simulink library "per"  (Simulink 8.2)
settings: Solver=ode45  StartTime=0.0  StopTime=10.0  RelTol=1e-3
undefined symbols (not defined in the file or in its folder): C_TICK_TIME_S, ENUM_LANEQUALITY_HIGH, ENUM_LANEQUALITY_MEDIUM, ENUM_SENSORSTATE_NORMAL, FALSE, KAPP_VehicleWidth_m, KPER_C0CrossingThr_m, KPER_CalDefaultTLC_s, KPER_CalTLCMax_s, KPER_CalTLCMin_s, KPER_DefaultLaneWidth_m, KPER_LaneWidHoldOnTime_s, KPER_LaneWidRampFinErrThres_m, KPER_LaneWidRampFinTimeThres_s, KPER_LaneWidRampInFalRt_mps, KPER_LaneWidRampInRisRt_mps, KPER_LaneWidRampOutFalRt_mps, KPER_LaneWidRampOutRisRt_mps, KPER_TLCDefaultValue_s, KPER_UseCalTLC_flg, TRUE
libraries: hcu_lib x16, cam x1, rad x1, sdf x1
(part 2 of 2)

== system per/PER/per/Lane_Process/LaneCalculation/GenerateRightLane ==
  VDINR_LaneC0R_m : Inport
  VPER_EstLaneC0R_m : Inport  Port=2
  VDINR_LaneC1R_rad : Inport  Port=3
  VPER_EstLaneC1R_rad : Inport  Port=4
  VDINR_LaneC2R_rat : Inport  Port=5
  VPER_EstLaneC2R_rat : Inport  Port=6
  VDINR_LaneC3R_rat : Inport  Port=7
  VPER_EstLaneC3R_rat : Inport  Port=8
  VPER_RightLaneAvail_flg : Inport  Port=9
  Switch{3,12..14} (4 alike) : Switch  Criteria=u2 ~= 0
  VPER_LaneC0R_m : Outport
  VPER_LaneC1R_rad : Outport  Port=2
  VPER_LaneC2R_rat : Outport  Port=3
  VPER_LaneC3R_rat : Outport  Port=4
  wires:
  VDINR_LaneC0R_m/1 -> Switch3/1
  VDINR_LaneC3R_rat/1 -> Switch14/1
  VPER_EstLaneC3R_rat/1 -> Switch14/3
  Switch14/1 -> VPER_LaneC3R_rat/1  "VPER_LaneC3R_rat"
  VPER_RightLaneAvail_flg/1 -> Switch3/2, Switch12/2, Switch13/2, Switch14/2
  VDINR_LaneC2R_rat/1 -> Switch13/1
  VPER_EstLaneC2R_rat/1 -> Switch13/3
  Switch13/1 -> VPER_LaneC2R_rat/1  "VPER_LaneC2R_rat"
  Switch3/1 -> VPER_LaneC0R_m/1  "VPER_LaneC0R_m"
  VDINR_LaneC1R_rad/1 -> Switch12/1
  VPER_EstLaneC1R_rad/1 -> Switch12/3
  Switch12/1 -> VPER_LaneC1R_rad/1  "VPER_LaneC1R_rad"
  VPER_EstLaneC0R_m/1 -> Switch3/3

== system per/PER/per/Lane_Process/LaneCalculation/LR_Available ==
  VDINR_LaneC0L_m : Inport
  VDINR_LaneC0R_m : Inport  Port=2
  VDINR_LaneC1L_rad : Inport  Port=3
  VDINR_LaneC1R_rad : Inport  Port=4
  VDINR_LaneC2L_rat : Inport  Port=5
  VDINR_LaneC2R_rat : Inport  Port=6
  VDINR_LaneC3L_rat : Inport  Port=7
  VDINR_LaneC3R_rat : Inport  Port=8
  Enable : EnablePort  StatesWhenEnabling=reset
  Add{,1..3} (4 alike) : Sum
  Gain{,1..3} (4 alike) : Gain  Gain=0.5
  VPER_RLCenterLineC0_m : Outport
  VPER_RLCenterLineC1_rad : Outport  Port=2
  VPER_RLCenterLineC2_rat : Outport  Port=3
  VPER_RLCenterLineC3_rat : Outport  Port=4
  wires:
  VDINR_LaneC0L_m/1 -> Add/1
  VDINR_LaneC0R_m/1 -> Add/2
  Add/1 -> Gain/1
  Gain/1 -> VPER_RLCenterLineC0_m/1  "VPER_RLCenterLineC0_m"
  VDINR_LaneC1L_rad/1 -> Add1/1
  VDINR_LaneC1R_rad/1 -> Add1/2
  Add1/1 -> Gain1/1
  Add2/1 -> Gain2/1
  Gain1/1 -> VPER_RLCenterLineC1_rad/1  "VPER_RLCenterLineC1_rad"
  VDINR_LaneC2L_rat/1 -> Add2/1
  VDINR_LaneC2R_rat/1 -> Add2/2
  Gain2/1 -> VPER_RLCenterLineC2_rat/1  "VPER_RLCenterLineC2_rat"
  Add3/1 -> Gain3/1
  VDINR_LaneC3L_rat/1 -> Add3/1
  VDINR_LaneC3R_rat/1 -> Add3/2
  Gain3/1 -> VPER_RLCenterLineC3_rat/1  "VPER_RLCenterLineC3_rat"

== system per/PER/per/Lane_Process/LaneCalculation/LR_NotAvailable ==
  VPER_EstLaneC0L_m : Inport
  VPER_EstLaneC0R_m : Inport  Port=2
  VPER_EstLaneC1L_rad : Inport  Port=3
  VPER_EstLaneC1R_rad : Inport  Port=4
  VPER_EstLaneC2L_rat : Inport  Port=5
  VPER_EstLaneC2R_rat : Inport  Port=6
  VPER_EstLaneC3L_rat : Inport  Port=7
  VPER_EstLaneC3R_rat : Inport  Port=8
  Enable : EnablePort  StatesWhenEnabling=reset
  Add{,1..3} (4 alike) : Sum
  Gain{,1..3} (4 alike) : Gain  Gain=0.5
  VPER_EstCenterLineC0_m : Outport
  VPER_EstCenterLineC1_rad : Outport  Port=2
  VPER_EstCenterLineC2_rat : Outport  Port=3
  VPER_EstCenterLineC3_rat : Outport  Port=4
  wires:
  VPER_EstLaneC0L_m/1 -> Add/1
  VPER_EstLaneC0R_m/1 -> Add/2
  Add/1 -> Gain/1
  Gain/1 -> VPER_EstCenterLineC0_m/1  "VPER_EstCenterLineC0_m"
  VPER_EstLaneC1L_rad/1 -> Add1/1
  VPER_EstLaneC1R_rad/1 -> Add1/2
  Add1/1 -> Gain1/1
  Add2/1 -> Gain2/1
  Gain1/1 -> VPER_EstCenterLineC1_rad/1  "VPER_EstCenterLineC1_rad"
  VPER_EstLaneC2L_rat/1 -> Add2/1
  VPER_EstLaneC2R_rat/1 -> Add2/2
  Gain2/1 -> VPER_EstCenterLineC2_rat/1  "VPER_EstCenterLineC2_rat"
  Add3/1 -> Gain3/1
  VPER_EstLaneC3L_rat/1 -> Add3/1
  VPER_EstLaneC3R_rat/1 -> Add3/2
  Gain3/1 -> VPER_EstCenterLineC3_rat/1  "VPER_EstCenterLineC3_rat"

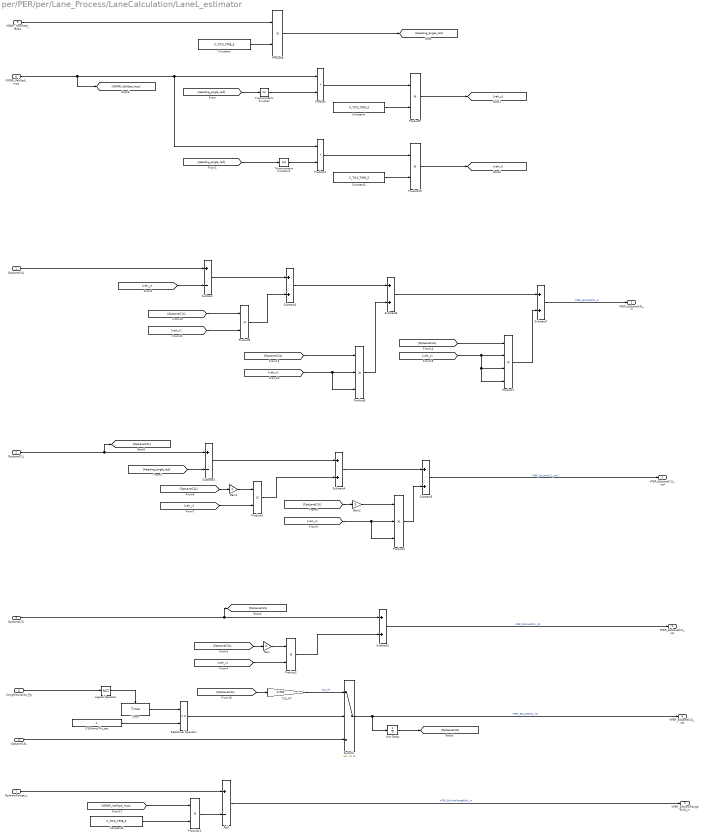
== system per/PER/per/Lane_Process/LaneCalculation/LaneL_estimator ==
  OptLaneC0L : Inport
  OptLaneC1L : Inport  Port=2
  OptLaneC2L : Inport  Port=3
  OptLaneC3L : Inport  Port=4
  VDINR_YawRate_radps : Inport  Port=5
  VDINR_VehSpd_mps : Inport  Port=6
  OptViewRange_L : Inport  Port=7
  UsingRawLaneL_flg : Inport  Port=8
  Add : Sum  Inputs=+-
  C3LRampThr_sec : Constant  OutDataTypeStr=single
  C3L_FF : Gain  Gain=0.994
  Constant{,1..2,4} (4 alike) : Constant  Value=C_TICK_TIME_S
  Gain : Gain  Gain=3
  Gain1 : Gain  Gain=2
  Gain2 : Gain  Gain=3
  Logical Operator : Logic  Operator=NOT  AllPortsSameDT=off  OutDataTypeStr=boolean
  Product{,1..3,5,8..10,12} (9 alike) : Product
  Product4 : Product  Inputs=3
  Product6 : Product  Inputs=3
  Product7 : Product  Inputs=4
  Relational Operator : RelationalOperator  OutDataTypeStr=boolean
  Subtract : Sum  Inputs=+-
  Subtract{1..2,4..7} (6 alike) : Sum
  Subtract3 : Sum  Inputs=+-
  Switch2 : Switch  Criteria=u2 ~= 0
  Timer : hcu_lib/Timer  SystemSampleTime=-1
  Trigonometric Function : Trigonometry
  Trigonometric Function1 : Trigonometry  Operator=cos
  Unit Delay : UnitDelay  SampleTime=-1
  VPER_EstLaneC0L_m : Outport
  VPER_EstLaneC1L_rad : Outport  Port=2
  VPER_EstLaneC2L_rat : Outport  Port=3
  VPER_EstLaneC3L_rat : Outport  Port=4
  VPER_EstViewRangeEndL_m : Outport  Port=5
  wires:
  VDINR_VehSpd_mps/1 -> [VDINR_VehSpd_mps], Product1/1, Product/1
  [Heading_angle_rad] -> Trigonometric Function/1
  Trigonometric Function/1 -> Product/2
  Product9/1 -> [veh_y]
  [Heading_angle_rad] -> Trigonometric Function1/1
  Trigonometric Function1/1 -> Product1/2
  Product10/1 -> [veh_x]
  OptLaneC0L/1 -> Subtract/1
  [veh_y] -> Subtract/2
  Subtract/1 -> Subtract1/1
  OptLaneC2L/1 -> [OptLaneC2L], Subtract2/1
  Product2/1 -> Subtract2/2
  [OptLaneC3L] -> Gain/1
  Gain/1 -> Product2/1
  [veh_x] -> Product2/2
  Subtract2/1 -> VPER_EstLaneC2L_rat/1  "VPER_EstLaneC2L_rat"
  OptLaneC1L/1 -> [OptLaneC1L], Subtract3/1
  [Heading_angle_rad] -> Subtract3/2
  Subtract3/1 -> Subtract4/1
  [OptLaneC2L] -> Gain1/1
  Gain1/1 -> Product3/1
  [veh_x] -> Product3/2
  Product3/1 -> Subtract4/2
  Subtract4/1 -> Subtract5/1
  [OptLaneC3L] -> Gain2/1
  Gain2/1 -> Product4/1
  [veh_x] -> Product4/3, Product4/2
  Product4/1 -> Subtract5/2
  Subtract5/1 -> VPER_EstLaneC1L_rad/1  "VPER_EstLaneC1L_rad"
  [OptLaneC1L] -> Product5/1
  [veh_x] -> Product5/2
  Product5/1 -> Subtract1/2
  Subtract1/1 -> Subtract6/1
  [OptLaneC2L] -> Product6/1
  [veh_x] -> Product6/2, Product6/3
  Product6/1 -> Subtract6/2
  Subtract6/1 -> Subtract7/1
  [OptLaneC3L] -> Product7/1
  [veh_x] -> Product7/2, Product7/4, Product7/3
  Product7/1 -> Subtract7/2
  Subtract7/1 -> VPER_EstLaneC0L_m/1  "VPER_EstLaneC0L_m"
  Constant/1 -> Product8/2
  Constant1/1 -> Product9/2
  Product/1 -> Product9/1
  Constant2/1 -> Product10/2
  Product1/1 -> Product10/1
  VDINR_YawRate_radps/1 -> Product8/1
  OptViewRange_L/1 -> Add/1
  [VDINR_VehSpd_mps] -> Product12/1
  Product12/1 -> Add/2
  Add/1 -> VPER_EstViewRangeEndL_m/1  "VPER_EstViewRangeEndL_m"
  Constant4/1 -> Product12/2
  UsingRawLaneL_flg/1 -> Logical Operator/1
  Timer/1 -> Relational Operator/1
  C3LRampThr_sec/1 -> Relational Operator/2
  Relational Operator/1 -> Switch2/2
  OptLaneC3L/1 -> Switch2/3
  Switch2/1 -> Unit Delay/1, VPER_EstLaneC3L_rat/1  "VPER_EstLaneC3L_rat"
  [OptLaneC3L] -> C3L_FF/1
  C3L_FF/1 -> Switch2/1  "C3L_FF"
  Logical Operator/1 -> Timer/Enable
  Unit Delay/1 -> [OptLaneC3L]
  Product8/1 -> [Heading_angle_rad]

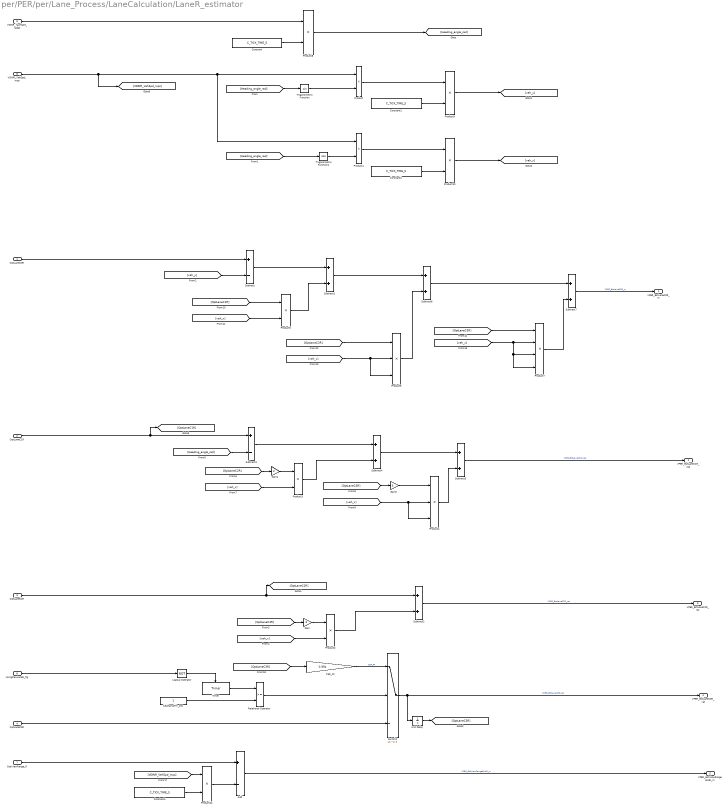
== system per/PER/per/Lane_Process/LaneCalculation/LaneR_estimator ==
  OptLaneC0R : Inport
  OptLaneC1R : Inport  Port=2
  OptLaneC2R : Inport  Port=3
  OptLaneC3R : Inport  Port=4
  VDINR_YawRate_radps : Inport  Port=5
  VDINR_VehSpd_mps : Inport  Port=6
  OptViewRange_R : Inport  Port=7
  UsingRawLaneR_flg : Inport  Port=8
  Add : Sum  Inputs=+-
  C3LRampThr_sec : Constant  OutDataTypeStr=single
  C3R_FF : Gain  Gain=0.994
  Constant{,1..2,4} (4 alike) : Constant  Value=C_TICK_TIME_S
  Gain : Gain  Gain=3
  Gain1 : Gain  Gain=2
  Gain2 : Gain  Gain=3
  Logical Operator : Logic  Operator=NOT  AllPortsSameDT=off  OutDataTypeStr=boolean
  Product{,1..3,5,8..10,12} (9 alike) : Product
  Product4 : Product  Inputs=3
  Product6 : Product  Inputs=3
  Product7 : Product  Inputs=4
  Relational Operator : RelationalOperator  OutDataTypeStr=boolean
  Subtract : Sum  Inputs=+-
  Subtract{1..2,4..7} (6 alike) : Sum
  Subtract3 : Sum  Inputs=+-
  Switch2 : Switch  Criteria=u2 ~= 0
  Timer : hcu_lib/Timer  SystemSampleTime=-1
  Trigonometric Function : Trigonometry
  Trigonometric Function1 : Trigonometry  Operator=cos
  Unit Delay : UnitDelay  SampleTime=-1
  VPER_EstLaneC0R_m : Outport
  VPER_EstLaneC1R_rad : Outport  Port=2
  VPER_EstLaneC2R_rat : Outport  Port=3
  VPER_EstLaneC3R_rat : Outport  Port=4
  VPER_EstViewRangeEndR_m : Outport  Port=5
  wires:
  Add/1 -> VPER_EstViewRangeEndR_m/1  "VPER_EstViewRangeEndR_m"
  Product12/1 -> Add/2
  Constant4/1 -> Product12/2
  [VDINR_VehSpd_mps] -> Product12/1
  OptViewRange_R/1 -> Add/1
  Product8/1 -> [Heading_angle_rad]
  VDINR_YawRate_radps/1 -> Product8/1
  Product1/1 -> Product10/1
  Constant2/1 -> Product10/2
  Product/1 -> Product9/1
  Constant1/1 -> Product9/2
  Constant/1 -> Product8/2
  Subtract7/1 -> VPER_EstLaneC0R_m/1  "VPER_EstLaneC0R_m"
  Product7/1 -> Subtract7/2
  [veh_x] -> Product7/3, Product7/4, Product7/2
  [OptLaneC3R] -> Product7/1
  Subtract6/1 -> Subtract7/1
  Product6/1 -> Subtract6/2
  [veh_x] -> Product6/3, Product6/2
  [OptLaneC2R] -> Product6/1
  Subtract1/1 -> Subtract6/1
  Product5/1 -> Subtract1/2
  [veh_x] -> Product5/2
  [OptLaneC1R] -> Product5/1
  Subtract5/1 -> VPER_EstLaneC1R_rad/1  "VPER_EstLaneC1R_rad"
  Product4/1 -> Subtract5/2
  [veh_x] -> Product4/2, Product4/3
  Gain2/1 -> Product4/1
  [OptLaneC3R] -> Gain2/1
  Subtract4/1 -> Subtract5/1
  Product3/1 -> Subtract4/2
  [veh_x] -> Product3/2
  Gain1/1 -> Product3/1
  [OptLaneC2R] -> Gain1/1
  Subtract3/1 -> Subtract4/1
  [Heading_angle_rad] -> Subtract3/2
  OptLaneC1R/1 -> Subtract3/1, [OptLaneC1R]
  Subtract2/1 -> VPER_EstLaneC2R_rat/1  "VPER_EstLaneC2R_rat"
  [veh_x] -> Product2/2
  Gain/1 -> Product2/1
  [OptLaneC3R] -> Gain/1
  Product2/1 -> Subtract2/2
  OptLaneC2R/1 -> Subtract2/1, [OptLaneC2R]
  Subtract/1 -> Subtract1/1
  [veh_y] -> Subtract/2
  OptLaneC0R/1 -> Subtract/1
  Product10/1 -> [veh_x]
  Trigonometric Function1/1 -> Product1/2
  [Heading_angle_rad] -> Trigonometric Function1/1
  Product9/1 -> [veh_y]
  Trigonometric Function/1 -> Product/2
  [Heading_angle_rad] -> Trigonometric Function/1
  VDINR_VehSpd_mps/1 -> Product/1, Product1/1, [VDINR_VehSpd_mps]
  UsingRawLaneR_flg/1 -> Logical Operator/1
  Timer/1 -> Relational Operator/1
  C3LRampThr_sec/1 -> Relational Operator/2
  Relational Operator/1 -> Switch2/2
  Switch2/1 -> Unit Delay/1, VPER_EstLaneC3R_rat/1  "VPER_EstLaneC3R_rat"
  [OptLaneC3R] -> C3R_FF/1
  C3R_FF/1 -> Switch2/1  "C3R_FF"
  OptLaneC3R/1 -> Switch2/3
  Logical Operator/1 -> Timer/Enable
  Unit Delay/1 -> [OptLaneC3R]

== system per/PER/per/Lane_Process/LaneCalculation/LaneResidual_Calculation ==
  VPER_EstViewRangeEndL_m : Inport
  VDINR_VehSpd_mps : Inport  Port=2
  VPER_EstViewRangeEndR_m : Inport  Port=3
  Constant6 : Constant  Value=3  OutDataTypeStr=single
  Constant7 : Constant  Value=3  OutDataTypeStr=single
  Saturation1 : Saturate  UpperLimit=3  LowerLimit=0
      settings: AttributesFormatString=upper = %<UpperLimit>\nlower = %<LowerLimit>
  Saturation2 : Saturate  UpperLimit=3  LowerLimit=0
      settings: AttributesFormatString=upper = %<UpperLimit>\nlower = %<LowerLimit>
  divide : hcu_lib/divide
  divide1 : hcu_lib/divide
  VPER_ResidualLaneL_s : Outport
  VPER_ResidualLaneR_s : Outport  Port=2
  wires:
  divide/1 -> Saturation1/1
  VPER_EstViewRangeEndL_m/1 -> divide/1
  Constant6/1 -> divide/3
  VPER_EstViewRangeEndR_m/1 -> divide1/1
  VDINR_VehSpd_mps/1 -> divide1/2, divide/2
  Constant7/1 -> divide1/3
  divide1/1 -> Saturation2/1
  Saturation1/1 -> VPER_ResidualLaneL_s/1  "VPER_ResidualLaneL_s"
  Saturation2/1 -> VPER_ResidualLaneR_s/1  "VPER_ResidualLaneR_s"

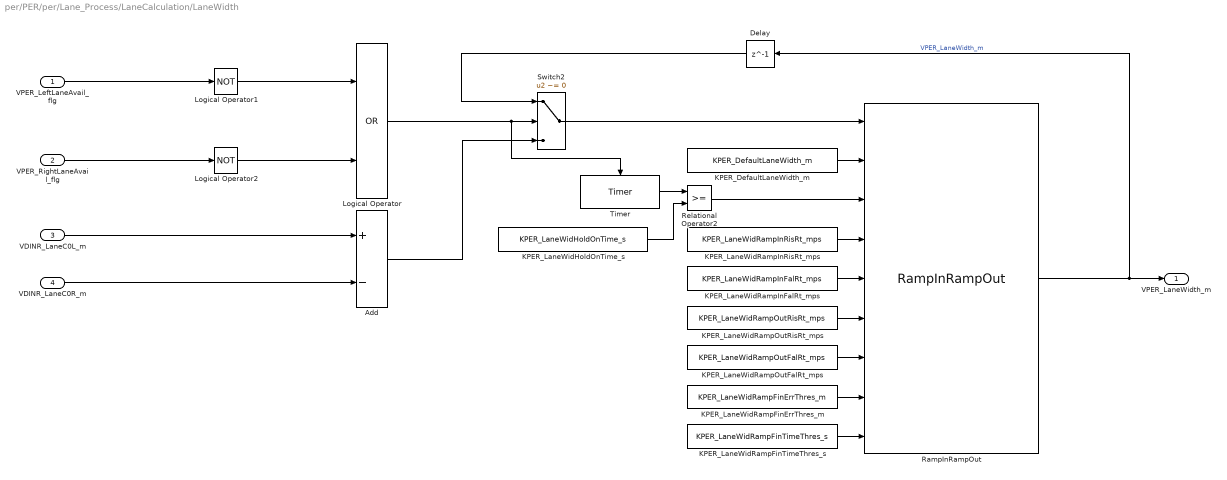
== system per/PER/per/Lane_Process/LaneCalculation/LaneWidth ==
  VPER_LeftLaneAvail_flg : Inport
  VPER_RightLaneAvail_flg : Inport  Port=2
  VDINR_LaneC0L_m : Inport  Port=3
  VDINR_LaneC0R_m : Inport  Port=4
  Add : Sum  Inputs=+-
  Delay : Delay  DelayLength=1  InitialCondition=KPER_DefaultLaneWidth_m
  KPER_DefaultLaneWidth_m : Constant  Value=KPER_DefaultLaneWidth_m
  KPER_LaneWidHoldOnTime_s : Constant  Value=KPER_LaneWidHoldOnTime_s
  KPER_LaneWidRampFinErrThres_m : Constant  Value=KPER_LaneWidRampFinErrThres_m
  KPER_LaneWidRampFinTimeThres_s : Constant  Value=KPER_LaneWidRampFinTimeThres_s
  KPER_LaneWidRampInFalRt_mps : Constant  Value=KPER_LaneWidRampInFalRt_mps
  KPER_LaneWidRampInRisRt_mps : Constant  Value=KPER_LaneWidRampInRisRt_mps
  KPER_LaneWidRampOutFalRt_mps : Constant  Value=KPER_LaneWidRampOutFalRt_mps
  KPER_LaneWidRampOutRisRt_mps : Constant  Value=KPER_LaneWidRampOutRisRt_mps
  Logical Operator : Logic  Operator=OR  AllPortsSameDT=off  OutDataTypeStr=boolean
  Logical Operator1 : Logic  Operator=NOT  AllPortsSameDT=off  OutDataTypeStr=boolean
  Logical Operator2 : Logic  Operator=NOT  AllPortsSameDT=off  OutDataTypeStr=boolean
  RampInRampOut : hcu_lib/RampInRampOut  SystemSampleTime=-1
  Relational Operator2 : RelationalOperator  OutDataTypeStr=boolean
  Switch2 : Switch  Criteria=u2 ~= 0
  Timer : hcu_lib/Timer  SystemSampleTime=-1
  VPER_LaneWidth_m : Outport
  wires:
  VDINR_LaneC0R_m/1 -> Add/2
  Add/1 -> Switch2/3
  VDINR_LaneC0L_m/1 -> Add/1
  Logical Operator2/1 -> Logical Operator/2
  Logical Operator1/1 -> Logical Operator/1
  Switch2/1 -> RampInRampOut/1
  Delay/1 -> Switch2/1
  KPER_DefaultLaneWidth_m/1 -> RampInRampOut/2
  Logical Operator/1 -> Switch2/2, Timer/Enable
  KPER_LaneWidRampInRisRt_mps/1 -> RampInRampOut/4
  KPER_LaneWidRampInFalRt_mps/1 -> RampInRampOut/5
  KPER_LaneWidRampOutFalRt_mps/1 -> RampInRampOut/7
  KPER_LaneWidRampOutRisRt_mps/1 -> RampInRampOut/6
  KPER_LaneWidRampFinErrThres_m/1 -> RampInRampOut/8
  KPER_LaneWidRampFinTimeThres_s/1 -> RampInRampOut/9
  RampInRampOut/1 -> Delay/1, VPER_LaneWidth_m/1  "VPER_LaneWidth_m"
  Relational Operator2/1 -> RampInRampOut/3
  Timer/1 -> Relational Operator2/1
  KPER_LaneWidHoldOnTime_s/1 -> Relational Operator2/2
  VPER_LeftLaneAvail_flg/1 -> Logical Operator1/1
  VPER_RightLaneAvail_flg/1 -> Logical Operator2/1

== system per/PER/per/Lane_Process/LaneCalculation/OnlyL_Available ==
  VPER_LaneWidth_m : Inport
  VDINR_LaneC0L_m : Inport  Port=2
  VDINR_LaneC1L_rad : Inport  Port=3
  VDINR_LaneC2L_rat : Inport  Port=4
  VDINR_LaneC3L_rat : Inport  Port=5
  Enable : EnablePort  StatesWhenEnabling=reset
  Add : Sum  Inputs=-+
  Add1 : Sum
  Data Type Conversion : DataTypeConversion  OutDataTypeStr=single
  Data Type Conversion1 : DataTypeConversion  OutDataTypeStr=single
  Data Type Conversion2 : DataTypeConversion  OutDataTypeStr=single
  Gain : Gain  Gain=0.5
  VPER_LCenterLineC0_m : Outport
  VPER_LCenterLineC1_rad : Outport  Port=2
  VPER_LCenterLineC2_rat : Outport  Port=3
  VPER_LCenterLineC3_rat : Outport  Port=4
  wires:
  VDINR_LaneC1L_rad/1 -> Data Type Conversion/1
  VPER_LaneWidth_m/1 -> Add/1
  VDINR_LaneC0L_m/1 -> Add1/2, Add/2
  VDINR_LaneC2L_rat/1 -> Data Type Conversion1/1
  VDINR_LaneC3L_rat/1 -> Data Type Conversion2/1
  Add/1 -> Add1/1
  Add1/1 -> Gain/1
  Gain/1 -> VPER_LCenterLineC0_m/1  "VPER_LCenterLineC0_m"
  Data Type Conversion1/1 -> VPER_LCenterLineC2_rat/1  "VPER_LCenterLineC2_rat"
  Data Type Conversion2/1 -> VPER_LCenterLineC3_rat/1  "VPER_LCenterLineC3_rat"
  Data Type Conversion/1 -> VPER_LCenterLineC1_rad/1  "VPER_LCenterLineC1_rad"

== system per/PER/per/Lane_Process/LaneCalculation/OnlyR_Available ==
  VPER_LaneWidth_m : Inport
  VDINR_LaneC0R_m : Inport  Port=2
  VDINR_LaneC1R_rad : Inport  Port=3
  VDINR_LaneC2R_rat : Inport  Port=4
  VDINR_LaneC3R_rat : Inport  Port=5
  Enable : EnablePort  StatesWhenEnabling=reset
  Add : Sum
  Add1 : Sum
  Data Type Conversion : DataTypeConversion  OutDataTypeStr=single
  Data Type Conversion1 : DataTypeConversion  OutDataTypeStr=single
  Data Type Conversion2 : DataTypeConversion  OutDataTypeStr=single
  Gain : Gain  Gain=0.5
  VPER_RCenterLineC0_m : Outport
  VPER_RCenterLineC1_rad : Outport  Port=2
  VPER_RCenterLineC2_rat : Outport  Port=3
  VPER_RCenterLineC3_rat : Outport  Port=4
  wires:
  VDINR_LaneC3R_rat/1 -> Data Type Conversion2/1
  VDINR_LaneC2R_rat/1 -> Data Type Conversion1/1
  VDINR_LaneC0R_m/1 -> Add1/2, Add/2
  VPER_LaneWidth_m/1 -> Add/1
  VDINR_LaneC1R_rad/1 -> Data Type Conversion/1
  Add/1 -> Add1/1
  Add1/1 -> Gain/1
  Gain/1 -> VPER_RCenterLineC0_m/1  "VPER_RCenterLineC0_m"
  Data Type Conversion/1 -> VPER_RCenterLineC1_rad/1  "VPER_RCenterLineC1_rad"
  Data Type Conversion1/1 -> VPER_RCenterLineC2_rat/1  "VPER_RCenterLineC2_rat"
  Data Type Conversion2/1 -> VPER_RCenterLineC3_rat/1  "VPER_RCenterLineC3_rat"

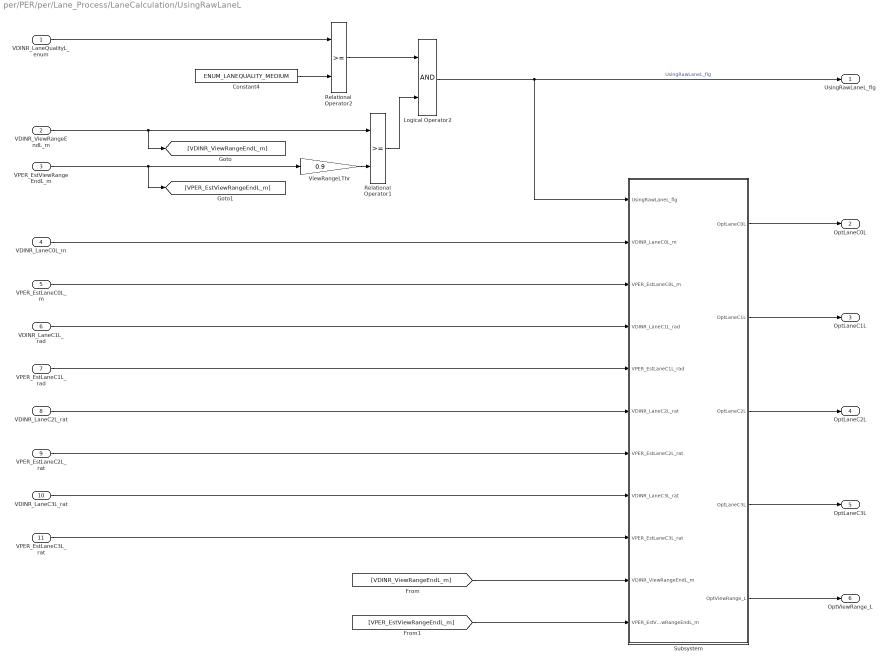
== system per/PER/per/Lane_Process/LaneCalculation/UsingRawLaneL ==
  VDINR_LaneQualityL_enum : Inport
  VDINR_ViewRangeEndL_m : Inport  Port=2
  VPER_EstViewRangeEndL_m : Inport  Port=3
  VDINR_LaneC0L_m : Inport  Port=4
  VPER_EstLaneC0L_m : Inport  Port=5
  VDINR_LaneC1L_rad : Inport  Port=6
  VPER_EstLaneC1L_rad : Inport  Port=7
  VDINR_LaneC2L_rat : Inport  Port=8
  VPER_EstLaneC2L_rat : Inport  Port=9
  VDINR_LaneC3L_rat : Inport  Port=10
  VPER_EstLaneC3L_rat : Inport  Port=11
  Constant4 : Constant  Value=ENUM_LANEQUALITY_MEDIUM
  Logical Operator2 : Logic  AllPortsSameDT=off  OutDataTypeStr=boolean
  Relational Operator1 : RelationalOperator  OutDataTypeStr=boolean
  Relational Operator2 : RelationalOperator  OutDataTypeStr=boolean
  Subsystem : Subsystem
  ViewRangeLThr : Gain  Gain=0.9
  UsingRawLaneL_flg : Outport
  OptLaneC0L : Outport  Port=2
  OptLaneC1L : Outport  Port=3
  OptLaneC2L : Outport  Port=4
  OptLaneC3L : Outport  Port=5
  OptViewRange_L : Outport  Port=6
  wires:
  Relational Operator1/1 -> Logical Operator2/2
  ViewRangeLThr/1 -> Relational Operator1/2
  VPER_EstViewRangeEndL_m/1 -> [VPER_EstViewRangeEndL_m], ViewRangeLThr/1
  VDINR_ViewRangeEndL_m/1 -> [VDINR_ViewRangeEndL_m], Relational Operator1/1
  Relational Operator2/1 -> Logical Operator2/1
  Constant4/1 -> Relational Operator2/2
  VDINR_LaneQualityL_enum/1 -> Relational Operator2/1
  Logical Operator2/1 -> Subsystem/1(UsingRawLaneL_flg), UsingRawLaneL_flg/1  "UsingRawLaneL_flg"
  VDINR_LaneC0L_m/1 -> Subsystem/2(VDINR_LaneC0L_m)
  VPER_EstLaneC0L_m/1 -> Subsystem/3(VPER_EstLaneC0L_m)
  VDINR_LaneC1L_rad/1 -> Subsystem/4(VDINR_LaneC1L_rad)
  VPER_EstLaneC1L_rad/1 -> Subsystem/5(VPER_EstLaneC1L_rad)
  VDINR_LaneC2L_rat/1 -> Subsystem/6(VDINR_LaneC2L_rat)
  VPER_EstLaneC2L_rat/1 -> Subsystem/7(VPER_EstLaneC2L_rat)
  VDINR_LaneC3L_rat/1 -> Subsystem/8(VDINR_LaneC3L_rat)
  VPER_EstLaneC3L_rat/1 -> Subsystem/9(VPER_EstLaneC3L_rat)
  [VPER_EstViewRangeEndL_m] -> Subsystem/11(VPER_EstViewRangeEndL_m)
  [VDINR_ViewRangeEndL_m] -> Subsystem/10(VDINR_ViewRangeEndL_m)
  Subsystem/1(OptLaneC0L) -> OptLaneC0L/1
  Subsystem/2(OptLaneC1L) -> OptLaneC1L/1
  Subsystem/3(OptLaneC2L) -> OptLaneC2L/1
  Subsystem/4(OptLaneC3L) -> OptLaneC3L/1
  Subsystem/5(OptViewRange_L) -> OptViewRange_L/1

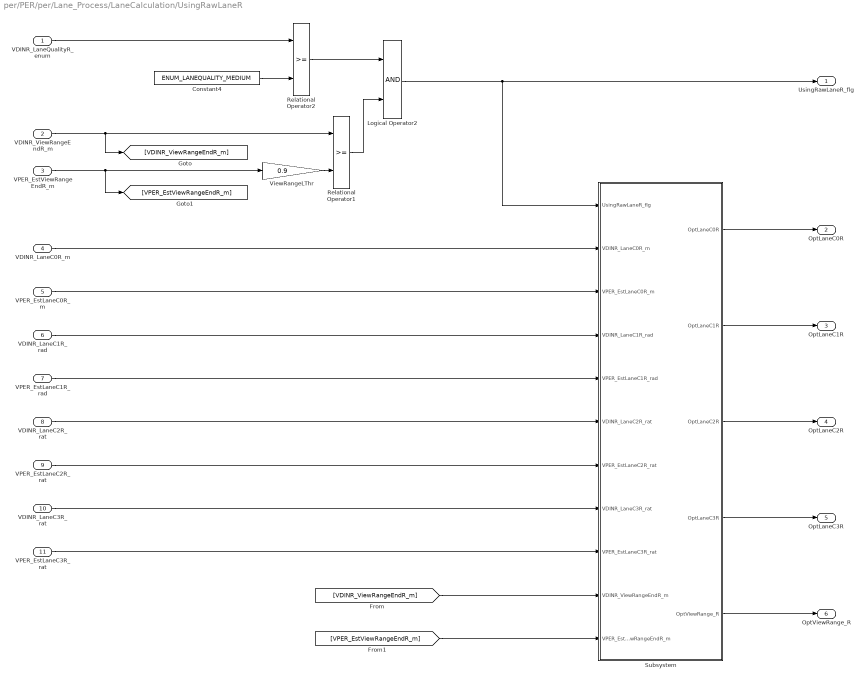
== system per/PER/per/Lane_Process/LaneCalculation/UsingRawLaneR ==
  VDINR_LaneQualityR_enum : Inport
  VDINR_ViewRangeEndR_m : Inport  Port=2
  VPER_EstViewRangeEndR_m : Inport  Port=3
  VDINR_LaneC0R_m : Inport  Port=4
  VPER_EstLaneC0R_m : Inport  Port=5
  VDINR_LaneC1R_rad : Inport  Port=6
  VPER_EstLaneC1R_rad : Inport  Port=7
  VDINR_LaneC2R_rat : Inport  Port=8
  VPER_EstLaneC2R_rat : Inport  Port=9
  VDINR_LaneC3R_rat : Inport  Port=10
  VPER_EstLaneC3R_rat : Inport  Port=11
  Constant4 : Constant  Value=ENUM_LANEQUALITY_MEDIUM
  Logical Operator2 : Logic  AllPortsSameDT=off  OutDataTypeStr=boolean
  Relational Operator1 : RelationalOperator  OutDataTypeStr=boolean
  Relational Operator2 : RelationalOperator  OutDataTypeStr=boolean
  Subsystem : Subsystem
  ViewRangeLThr : Gain  Gain=0.9
  UsingRawLaneR_flg : Outport
  OptLaneC0R : Outport  Port=2
  OptLaneC1R : Outport  Port=3
  OptLaneC2R : Outport  Port=4
  OptLaneC3R : Outport  Port=5
  OptViewRange_R : Outport  Port=6
  wires:
  Relational Operator1/1 -> Logical Operator2/2
  ViewRangeLThr/1 -> Relational Operator1/2
  VPER_EstViewRangeEndR_m/1 -> [VPER_EstViewRangeEndR_m], ViewRangeLThr/1
  VDINR_ViewRangeEndR_m/1 -> [VDINR_ViewRangeEndR_m], Relational Operator1/1
  Relational Operator2/1 -> Logical Operator2/1
  Constant4/1 -> Relational Operator2/2
  VDINR_LaneQualityR_enum/1 -> Relational Operator2/1
  Logical Operator2/1 -> Subsystem/1(UsingRawLaneR_flg), UsingRawLaneR_flg/1
  VDINR_LaneC0R_m/1 -> Subsystem/2(VDINR_LaneC0R_m)
  VPER_EstLaneC0R_m/1 -> Subsystem/3(VPER_EstLaneC0R_m)
  VDINR_LaneC1R_rad/1 -> Subsystem/4(VDINR_LaneC1R_rad)
  VPER_EstLaneC1R_rad/1 -> Subsystem/5(VPER_EstLaneC1R_rad)
  VDINR_LaneC2R_rat/1 -> Subsystem/6(VDINR_LaneC2R_rat)
  VPER_EstLaneC2R_rat/1 -> Subsystem/7(VPER_EstLaneC2R_rat)
  VDINR_LaneC3R_rat/1 -> Subsystem/8(VDINR_LaneC3R_rat)
  VPER_EstLaneC3R_rat/1 -> Subsystem/9(VPER_EstLaneC3R_rat)
  [VPER_EstViewRangeEndR_m] -> Subsystem/11(VPER_EstViewRangeEndR_m)
  [VDINR_ViewRangeEndR_m] -> Subsystem/10(VDINR_ViewRangeEndR_m)
  Subsystem/1(OptLaneC0R) -> OptLaneC0R/1
  Subsystem/2(OptLaneC1R) -> OptLaneC1R/1
  Subsystem/3(OptLaneC2R) -> OptLaneC2R/1
  Subsystem/4(OptLaneC3R) -> OptLaneC3R/1
  Subsystem/5(OptViewRange_R) -> OptViewRange_R/1

== system per/PER/per/Lane_Process/LaneCalculation/Using_estimator_LeftLane ==
  VDINR_LaneQualityL_enum : Inport
  VDINR_ViewRangeEndL_m : Inport  Port=2
  VPER_EstViewRangeEndL_m : Inport  Port=3
  Constant6 : Constant  Value=ENUM_LANEQUALITY_MEDIUM
  Logical Operator4 : Logic  AllPortsSameDT=off  OutDataTypeStr=boolean
  Relational Operator5 : RelationalOperator  OutDataTypeStr=boolean
  Relational Operator6 : RelationalOperator  OutDataTypeStr=boolean
  ViewRangeL : Gain  Gain=0.5
  VPER_LeftLaneAvail_flg : Outport
  wires:
  Relational Operator6/1 -> Logical Operator4/1
  Logical Operator4/1 -> VPER_LeftLaneAvail_flg/1  "VPER_LeftLaneAvail_flg"
  ViewRangeL/1 -> Relational Operator5/2
  Relational Operator5/1 -> Logical Operator4/2  "VRTiming_L"
  VPER_EstViewRangeEndL_m/1 -> ViewRangeL/1
  VDINR_LaneQualityL_enum/1 -> Relational Operator6/1
  Constant6/1 -> Relational Operator6/2
  VDINR_ViewRangeEndL_m/1 -> Relational Operator5/1

== system per/PER/per/Lane_Process/LaneCalculation/Using_estimator_RightLane ==
  VDINR_LaneQualityR_enum : Inport
  VDINR_ViewRangeEndR_m : Inport  Port=2
  VPER_EstViewRangeEndR_m : Inport  Port=3
  Constant7 : Constant  Value=ENUM_LANEQUALITY_MEDIUM
  Logical Operator5 : Logic  AllPortsSameDT=off  OutDataTypeStr=boolean
  Relational Operator7 : RelationalOperator  OutDataTypeStr=boolean
  Relational Operator8 : RelationalOperator  OutDataTypeStr=boolean
  ViewRangeR : Gain  Gain=0.5
  VPER_RightLaneAvail_flg : Outport
  wires:
  VDINR_ViewRangeEndR_m/1 -> Relational Operator7/1
  ViewRangeR/1 -> Relational Operator7/2
  VDINR_LaneQualityR_enum/1 -> Relational Operator8/1
  Constant7/1 -> Relational Operator8/2
  VPER_EstViewRangeEndR_m/1 -> ViewRangeR/1
  Relational Operator7/1 -> Logical Operator5/2  "VRTiming_R"
  Relational Operator8/1 -> Logical Operator5/1
  Logical Operator5/1 -> VPER_RightLaneAvail_flg/1  "VPER_RightLaneAvail_flg"

== system per/PER/per/Lane_Process/LaneCalculation/UsingRawLaneL/Subsystem ==
  UsingRawLaneL_flg : Inport
  VDINR_LaneC0L_m : Inport  Port=2
  VPER_EstLaneC0L_m : Inport  Port=3
  VDINR_LaneC1L_rad : Inport  Port=4
  VPER_EstLaneC1L_rad : Inport  Port=5
  VDINR_LaneC2L_rat : Inport  Port=6
  VPER_EstLaneC2L_rat : Inport  Port=7
  VDINR_LaneC3L_rat : Inport  Port=8
  VPER_EstLaneC3L_rat : Inport  Port=9
  VDINR_ViewRangeEndL_m : Inport  Port=10
  VPER_EstViewRangeEndL_m : Inport  Port=11
  Switch{1,4..7} (5 alike) : Switch  Criteria=u2 ~= 0
  OptLaneC0L : Outport
  OptLaneC1L : Outport  Port=2
  OptLaneC2L : Outport  Port=3
  OptLaneC3L : Outport  Port=4
  OptViewRange_L : Outport  Port=5
  wires:
  Switch1/1 -> OptViewRange_L/1  "OptViewRange_L"
  VPER_EstViewRangeEndL_m/1 -> Switch1/3
  UsingRawLaneL_flg/1 -> Switch5/2, Switch1/2, Switch7/2, Switch6/2, Switch4/2
  VDINR_ViewRangeEndL_m/1 -> Switch1/1
  Switch5/1 -> OptLaneC1L/1  "OptLaneC1L"
  Switch4/1 -> OptLaneC0L/1  "OptLaneC0L"
  Switch7/1 -> OptLaneC3L/1  "OptLaneC3L"
  VPER_EstLaneC3L_rat/1 -> Switch7/3
  VDINR_LaneC3L_rat/1 -> Switch7/1
  Switch6/1 -> OptLaneC2L/1  "OptLaneC2L"
  VPER_EstLaneC2L_rat/1 -> Switch6/3
  VDINR_LaneC2L_rat/1 -> Switch6/1
  VPER_EstLaneC1L_rad/1 -> Switch5/3
  VDINR_LaneC1L_rad/1 -> Switch5/1
  VPER_EstLaneC0L_m/1 -> Switch4/3
  VDINR_LaneC0L_m/1 -> Switch4/1

== system per/PER/per/Lane_Process/LaneCalculation/UsingRawLaneR/Subsystem ==
  UsingRawLaneR_flg : Inport
  VDINR_LaneC0R_m : Inport  Port=2
  VPER_EstLaneC0R_m : Inport  Port=3
  VDINR_LaneC1R_rad : Inport  Port=4
  VPER_EstLaneC1R_rad : Inport  Port=5
  VDINR_LaneC2R_rat : Inport  Port=6
  VPER_EstLaneC2R_rat : Inport  Port=7
  VDINR_LaneC3R_rat : Inport  Port=8
  VPER_EstLaneC3R_rat : Inport  Port=9
  VDINR_ViewRangeEndR_m : Inport  Port=10
  VPER_EstViewRangeEndR_m : Inport  Port=11
  Switch{1,4..7} (5 alike) : Switch  Criteria=u2 ~= 0
  OptLaneC0R : Outport
  OptLaneC1R : Outport  Port=2
  OptLaneC2R : Outport  Port=3
  OptLaneC3R : Outport  Port=4
  OptViewRange_R : Outport  Port=5
  wires:
  Switch1/1 -> OptViewRange_R/1  "OptViewRange_R"
  VPER_EstViewRangeEndR_m/1 -> Switch1/3
  UsingRawLaneR_flg/1 -> Switch5/2, Switch1/2, Switch7/2, Switch6/2, Switch4/2
  VDINR_ViewRangeEndR_m/1 -> Switch1/1
  Switch5/1 -> OptLaneC1R/1  "OptLaneC1R"
  Switch4/1 -> OptLaneC0R/1  "OptLaneC0R"
  Switch7/1 -> OptLaneC3R/1  "OptLaneC3R"
  VPER_EstLaneC3R_rat/1 -> Switch7/3
  VDINR_LaneC3R_rat/1 -> Switch7/1
  Switch6/1 -> OptLaneC2R/1  "OptLaneC2R"
  VPER_EstLaneC2R_rat/1 -> Switch6/3
  VDINR_LaneC2R_rat/1 -> Switch6/1
  VPER_EstLaneC1R_rad/1 -> Switch5/3
  VDINR_LaneC1R_rad/1 -> Switch5/1
  VPER_EstLaneC0R_m/1 -> Switch4/3
  VDINR_LaneC0R_m/1 -> Switch4/1

== stateflow chart PER/per/Lane_Process/LaneCalculation/Lane_status ==
  (default) -> (junction 13)
  (junction 13) -> (junction 14) [order 1] : [VPER_LeftLaneAvail_fig && VPER_RightLaneAvail_fig]
  (junction 13) -> (junction 15) [order 2]
  (junction 14) -> (junction 22) : {SWCase=1;
      | LR_avail=TRUE;
      | R_avail=FALSE;
      | L_avail=FALSE;
      | NO_avail=FALSE;}
  (junction 15) -> (junction 16) [order 1] : [(!VPER_C2Diff_flg || !VPER_LeftLaneAvail_fig) && VPER_RightLaneAvail_fig]
  (junction 15) -> (junction 17) [order 2]
  (junction 16) -> (junction 21) : {SWCase=2;
      | LR_avail=FALSE;
      | R_avail=TRUE;
      | L_avail=FALSE;
      | NO_avail=FALSE;}
  (junction 17) -> (junction 18) [order 1] : [VPER_LeftLaneAvail_fig && (VPER_C2Diff_flg || !VPER_RightLaneAvail_fig)]
  (junction 17) -> (junction 19) [order 2] : {SWCase=4;
      | LR_avail=FALSE;
      | R_avail=FALSE;
      | L_avail=FALSE;
      | NO_avail=TRUE;}
  (junction 18) -> (junction 20) : {SWCase=3;
      | LR_avail=FALSE;
      | R_avail=FALSE;
      | L_avail=TRUE;
      | NO_avail=FALSE;}
  (junction 20) -> (junction 19)
  (junction 21) -> (junction 20)
  (junction 22) -> (junction 21)
  data: VPER_LeftLaneAvail_fig input double; VPER_RightLaneAvail_fig input double; SWCase output single; LR_avail output boolean; R_avail output boolean; L_avail output boolean; NO_avail output boolean; TRUE parameter double; FALSE parameter double; VPER_C2Diff_flg input double

== stateflow chart PER/per/Lane_Process/C1R_Bias/Forgetting_factor/FF ==
  state Forget_Factor
    (default) -> (junction 39) : {P=1;
        | C1RBias_new_store = C1RBias_new;
        | P_R = P;
        | C1R_Bias = C1RBias_new_store;}
    Forget_Factor -> (junction 39)
    (junction 39) -> (junction 40) : {C1RBias_new_store = C1RBias_new_store + P*(C1RBias_new - C1RBias_new_store)/(Forget_Factor+P);
        | P = (P-P*P/(Forget_Factor+P))/Forget_Factor;
        | P_R=P;
        | C1R_Bias=C1RBias_new_store;}
  data: C1RBias_new input single; P local single; C1RBias_new_store local single; Forget_Factor input single; C1R_Bias output single; P_R output single

== stateflow chart PER/per/Lane_Process/C1L_Bias/Forgetting_factor/FF ==
  state Forget_Factor
    (default) -> (junction 53) : {P=1;
        | C1LBias_new_store = C1LBias_new;
        | P_L = P;
        | C1L_Bias = C1LBias_new_store;}
    Forget_Factor -> (junction 53)
    (junction 53) -> (junction 54) : {C1LBias_new_store = C1LBias_new_store + P*(C1LBias_new - C1LBias_new_store)/(Forget_Factor+P);
        | P = (P-P*P/(Forget_Factor+P))/Forget_Factor;
        | P_L=P;
        | C1L_Bias=C1LBias_new_store;}
  data: C1LBias_new input single; P local single; C1LBias_new_store local single; Forget_Factor input single; C1L_Bias output single; P_L output single
